simulink model "Assertion_TestGen5"  (R2017b)
settings: Solver=FixedStepDiscrete  StartTime=0.0  StopTime=10.0  RelTol=1e-3
undefined symbols (not defined in the file): Block_TestLib, reset
settings Model: Creator=hbourbou  LastModifiedBy=hbourbou
settings DebuggingCC: ParameterOverflowMsg=none

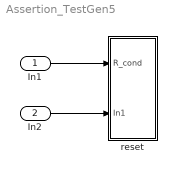
== system Assertion_TestGen5 ==
  In1 : Inport
  In2 : Inport  Port=2
  reset : Subsystem  AncestorBlock=Block_TestLib/reset
  wires:
  In1/1 -> reset/1(R_cond)
  In2/1 -> reset/2(In1)

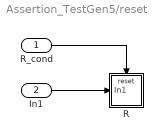
== system Assertion_TestGen5/reset ==
  R_cond : Inport  OutDataTypeStr=boolean
  In1 : Inport  Port=2
  R : Subsystem  TreatAsAtomicUnit=on
  wires:
  R_cond/1 -> R/Reset
  In1/1 -> R/1(In1)

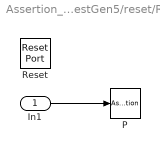
== system Assertion_TestGen5/reset/R ==
  In1 : Inport  OutDataTypeStr=int16  PortDimensions=[2,3]
  Reset : ResetPort  DisableCoverage=on
  P : Assertion  StopWhenAssertionFail=off
  wires:
  In1/1 -> P/1
